simulink model "track_kf_sim"  (R2017a)
settings: Solver=VariableStepAuto  StartTime=0.0  StopTime=100.0  RelTol=1e-3
libraries: simulink x2
settings Model: Creator=cg  LastModifiedBy=cg

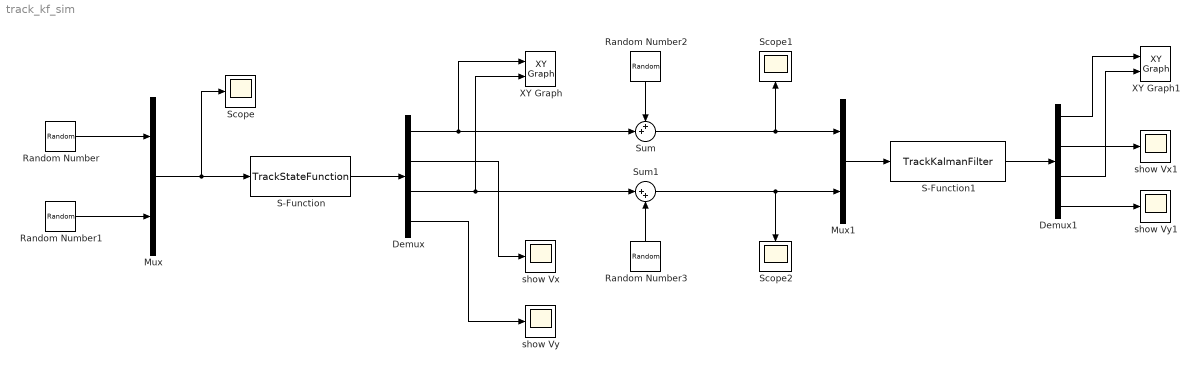
== system track_kf_sim ==
  Demux : Demux
  Demux1 : Demux
  Mux : Mux  Inputs=2
  Mux1 : Mux  Inputs=2
  Random Number : RandomNumber  Variance=0.0001  SampleTime=1
  Random Number1 : RandomNumber  Variance=0.0009  Seed=3  SampleTime=1
  Random Number2 : RandomNumber  Variance=0.04  SampleTime=1
  Random Number3 : RandomNumber  Variance=0.04  SampleTime=1
  S-Function : S-Function  FunctionName=TrackStateFunction  SFunctionDeploymentMode=off  EnableBusSupport=off
  S-Function1 : S-Function  FunctionName=TrackKalmanFilter  SFunctionDeploymentMode=off  EnableBusSupport=off
  Scope : Scope
  Scope1 : Scope
  Scope2 : Scope
  Sum : Sum  Inputs=++|
  Sum1 : Sum  Inputs=|++
  XY Graph : simulink/Sinks/XY Graph  xmin=0  xmax=600  ymin=0  ymax=600  st=1
  XY Graph1 : simulink/Sinks/XY Graph  xmin=0  xmax=600  ymin=0  ymax=600  st=1
  show Vx : Scope
  show Vx1 : Scope
  show Vy : Scope
  show Vy1 : Scope
  wires:
  Random Number/1 -> Mux/1
  Random Number1/1 -> Mux/2
  Mux/1 -> Scope/1, S-Function/1
  S-Function/1 -> Demux/1
  Demux/1 -> Sum/2, XY Graph/1
  Demux/3 -> Sum1/1, XY Graph/2
  Demux/2 -> show Vx/1
  Demux/4 -> show Vy/1
  Random Number2/1 -> Sum/1
  Random Number3/1 -> Sum1/2
  Sum/1 -> Scope1/1, Mux1/1
  Sum1/1 -> Scope2/1, Mux1/2
  Mux1/1 -> S-Function1/1
  S-Function1/1 -> Demux1/1
  Demux1/2 -> show Vx1/1
  Demux1/4 -> show Vy1/1
  Demux1/1 -> XY Graph1/1
  Demux1/3 -> XY Graph1/2
